simulink model "fifth_custom_ckt"  (R2018a)
settings: Solver=VariableStepAuto  StartTime=0.0  StopTime=10.0  RelTol=1e-3
settings Model: Creator=Gideon  LastModifiedBy=Gideon

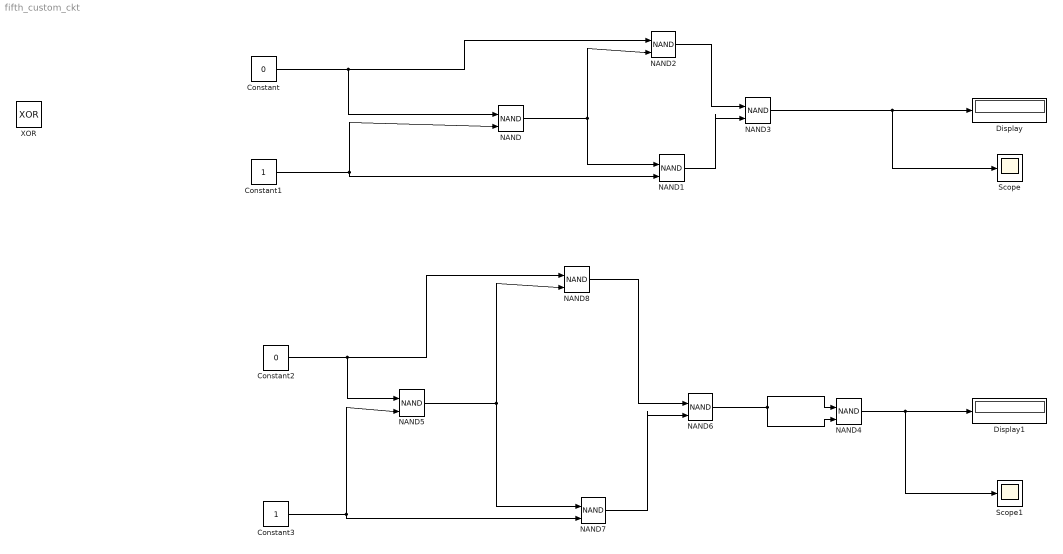
== system fifth_custom_ckt ==
  Constant : Constant  Value=0
  Constant1 : Constant
  Constant2 : Constant  Value=0
  Constant3 : Constant
  Display : Display
  Display1 : Display
  NAND{,1..8} (9 alike) : Logic  Operator=NAND  IconShape=distinctive  AllPortsSameDT=off  OutDataTypeStr=boolean
  Scope : Scope
  Scope1 : Scope
  XOR : Logic  Operator=XOR  IconShape=distinctive  AllPortsSameDT=off  OutDataTypeStr=boolean
  wires:
  Constant/1 -> NAND/1, NAND2/1
  Constant1/1 -> NAND/2, NAND1/2
  NAND/1 -> NAND1/1, NAND2/2
  NAND1/1 -> NAND3/2
  NAND2/1 -> NAND3/1
  NAND3/1 -> Scope/1, Display/1
  NAND4/1 -> Scope1/1, Display1/1
  Constant2/1 -> NAND5/1, NAND8/1
  Constant3/1 -> NAND5/2, NAND7/2
  NAND5/1 -> NAND7/1, NAND8/2
  NAND7/1 -> NAND6/2
  NAND8/1 -> NAND6/1
  NAND6/1 -> NAND4/2, NAND4/1
